simulink model "antisloshing_robot"  (R2025b)
settings: Solver=VariableStepAuto  StartTime=0.0  StopTime=10.0  RelTol=1e-3
undefined symbols (not defined in the file or in its folder): A_mat, B_full, K_mat

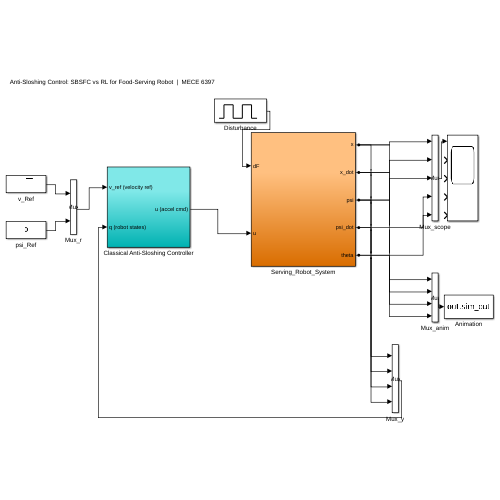
[thumbnail: Simulink's stored preview of the top-level diagram]
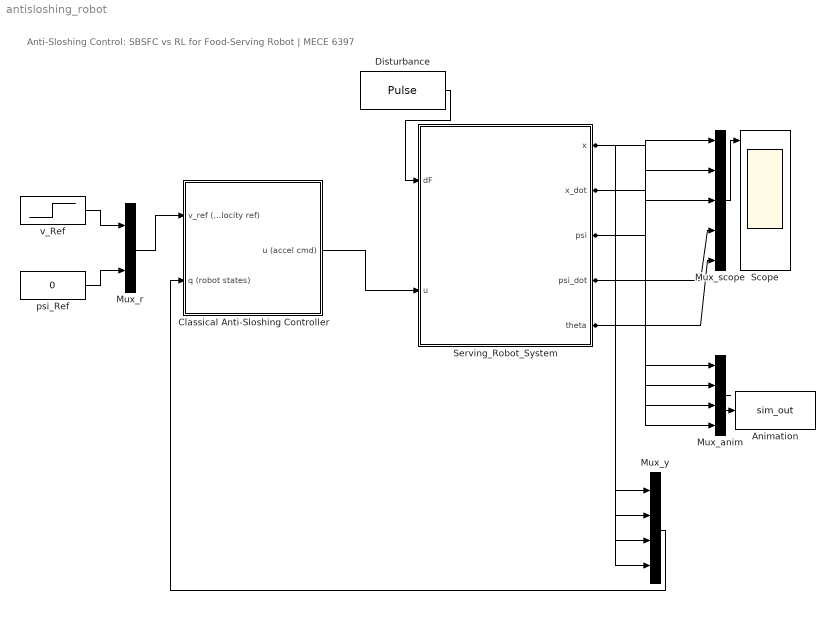
== system antisloshing_robot ==
  note: Anti-Sloshing Control: SBSFC vs RL for Food-Serving Robot | MECE 6397
  Animation : ToWorkspace  VariableName=sim_out  SaveFormat=Timeseries  SampleTime=-1
  Classical Anti-Sloshing Controller : Subsystem
  Disturbance : DiscretePulseGenerator  PulseType=Time based  Amplitude=15  Period=10  PulseWidth=10  PhaseDelay=5
  Mux_anim : Mux
  Mux_r : Mux  Inputs=2
  Mux_scope : Mux  Inputs=5
  Mux_y : Mux
  Scope : Scope  NumInputPorts=5
  Serving_Robot_System : Subsystem
  psi_Ref : Constant  Value=0
  v_Ref : Step  After=0.5  SampleTime=0
  wires:
  v_Ref/1 -> Mux_r/1
  psi_Ref/1 -> Mux_r/2
  Mux_r/1 -> Classical Anti-Sloshing Controller/1(v_ref (velocity ref))
  Disturbance/1 -> Serving_Robot_System/1(dF)
  Classical Anti-Sloshing Controller/1(u (accel cmd)) -> Serving_Robot_System/2(u)
  Serving_Robot_System/1(x) -> Mux_scope/1, Mux_y/1, Mux_anim/1
  Serving_Robot_System/2(x_dot) -> Mux_scope/2, Mux_y/2, Mux_anim/4
  Serving_Robot_System/3(psi) -> Mux_scope/3, Mux_y/3, Mux_anim/2
  Serving_Robot_System/4(psi_dot) -> Mux_scope/4, Mux_y/4
  Serving_Robot_System/5(theta) -> Mux_scope/5, Mux_anim/3
  Mux_scope/1 -> Scope/1
  Mux_y/1 -> Classical Anti-Sloshing Controller/2(q (robot states))
  Mux_anim/1 -> Animation/1

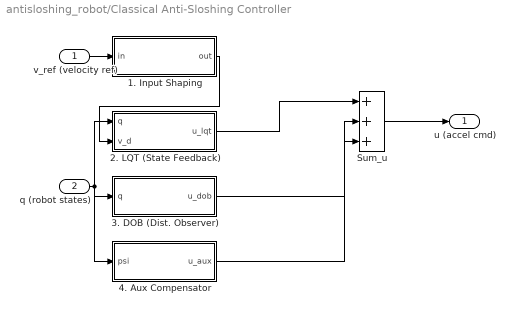
== system antisloshing_robot/Classical Anti-Sloshing Controller ==
  v_ref (velocity ref) : Inport
  q (robot states) : Inport  Port=2
  1. Input Shaping : Subsystem
  2. LQT (State Feedback) : Subsystem
  3. DOB (Dist. Observer) : Subsystem
  4. Aux Compensator : Subsystem
  Sum_u : Sum  Inputs=+++
  u (accel cmd) : Outport
  wires:
  v_ref (velocity ref)/1 -> 1. Input Shaping/1(in)
  1. Input Shaping/1(out) -> 2. LQT (State Feedback)/2(v_d)
  q (robot states)/1 -> 2. LQT (State Feedback)/1(q), 3. DOB (Dist. Observer)/1(q), 4. Aux Compensator/1(psi)
  2. LQT (State Feedback)/1(u_lqt) -> Sum_u/1
  3. DOB (Dist. Observer)/1(u_dob) -> Sum_u/2
  4. Aux Compensator/1(u_aux) -> Sum_u/3
  Sum_u/1 -> u (accel cmd)/1

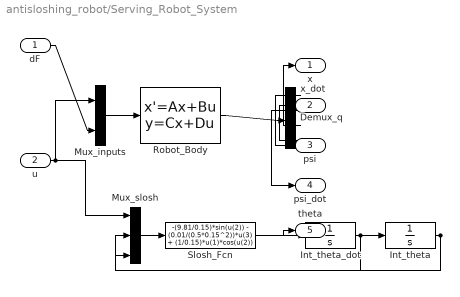
== system antisloshing_robot/Serving_Robot_System ==
  dF : Inport
  u : Inport  Port=2
  Demux_q : Demux
  Int_theta : Integrator
  Int_theta_dot : Integrator
  Mux_inputs : Mux  Inputs=2
  Mux_slosh : Mux  Inputs=3
  Robot_Body : StateSpace  A=A_mat  B=B_full  C=eye(4)  D=zeros(4,2)  InitialCondition=zeros(4,1)
  Slosh_Fcn : Fcn  Expr=-(9.81/0.15)*sin(u(2)) - (0.01/(0.5*0.15^2))*u(3) + (1/0.15)*u(1)*cos(u(2))
  x : Outport
  x_dot : Outport  Port=2
  psi : Outport  Port=3
  psi_dot : Outport  Port=4
  theta : Outport  Port=5
  wires:
  u/1 -> Mux_inputs/1, Mux_slosh/1
  dF/1 -> Mux_inputs/2
  Mux_inputs/1 -> Robot_Body/1
  Robot_Body/1 -> Demux_q/1
  Demux_q/3 -> x/1
  Demux_q/4 -> x_dot/1
  Demux_q/1 -> psi/1
  Demux_q/2 -> psi_dot/1
  Mux_slosh/1 -> Slosh_Fcn/1
  Slosh_Fcn/1 -> Int_theta_dot/1
  Int_theta_dot/1 -> Int_theta/1, Mux_slosh/3
  Int_theta/1 -> theta/1, Mux_slosh/2

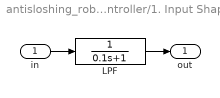
== system antisloshing_robot/Classical Anti-Sloshing Controller/1. Input Shaping ==
  in : Inport
  LPF : TransferFcn  Denominator=[0.1 1]
  out : Outport
  wires:
  in/1 -> LPF/1
  LPF/1 -> out/1

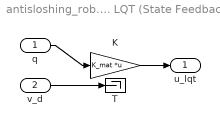
== system antisloshing_robot/Classical Anti-Sloshing Controller/2. LQT (State Feedback) ==
  q : Inport
  v_d : Inport  Port=2
  K : Gain  Gain=K_mat  Multiplication=Matrix(K*u)
  T : Terminator
  u_lqt : Outport
  wires:
  q/1 -> K/1
  K/1 -> u_lqt/1
  v_d/1 -> T/1

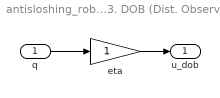
== system antisloshing_robot/Classical Anti-Sloshing Controller/3. DOB (Dist. Observer) ==
  q : Inport
  eta : Gain
  u_dob : Outport
  wires:
  q/1 -> eta/1
  eta/1 -> u_dob/1

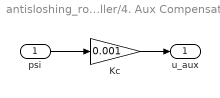
== system antisloshing_robot/Classical Anti-Sloshing Controller/4. Aux Compensator ==
  psi : Inport
  Kc : Gain  Gain=0.001
  u_aux : Outport
  wires:
  psi/1 -> Kc/1
  Kc/1 -> u_aux/1
